simulink model "three_phase_motor"  (R2018a)
settings: Solver=VariableStepDiscrete  StartTime=0.0  StopTime=2  RelTol=1e-3
values from neighbouring files (symbols this model uses):
  Ts = 0.0001    [pump_ori_perf.mat]
libraries: powerlib x2, powerlib_meascontrol x2, electricdrivelib x1
settings Model: Creator=siwak  LastModifiedBy=siwak

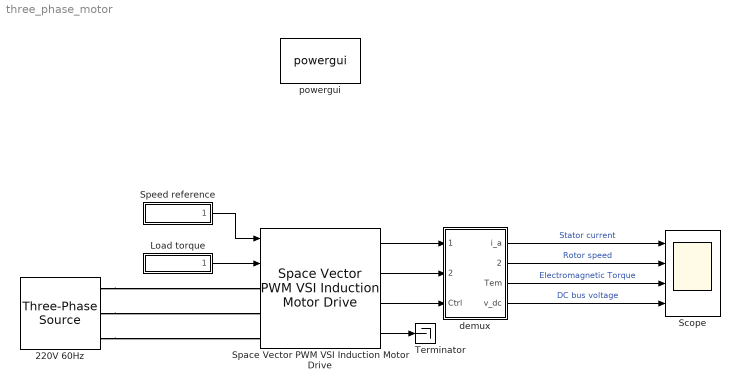
== system three_phase_motor ==
  220V 60Hz : powerlib/Electrical Sources/Three-Phase Source  InternalConnection=Yg  VoltagePhases=off  Voltage=220  PhaseAngle=0  Voltage_phases=[25e3 25e3 25e3]/sqrt(3)  PhaseAngles_phases=[0 -120 +120]  Frequency=60  NonIdealSource=on  SpecifyImpedance=off  Resistance=0.02  Inductance=0.05e-3  ShortCircuitLevel=100e6  BaseVoltage=25e3  XRratio=7  BusType=swing  Pref=0  Qref=0  Prefabc=[10e3, 10e3, 10e3]  Qrefabc=[0, 0, 0]  Qmin=-inf  Qmax=inf
  Load torque : Subsystem
  Scope : Scope  NumInputPorts=4
  Space Vector PWM VSI Induction Motor Drive : electricdrivelib/AC drives/Space Vector PWM VSI Induction Motor Drive  ReferenceFrame=Stationary  IterativeDiscreteModel=Trapezoidal non iterative  Pn=2238  Vn=220  fn=60  Rs=0.435  Lls=0.002  Lms=69.31e-3  Rr=0.816  Llr=0.002  ia=0  pha=0  ib=0  phb=0  ic=0  phc=0  J=0.089  Friction=0.005  p=2  slip=1  thdeg=0  Rsnb_rec=10e3  Csnb_rec=20e-9  Ron_rec=1e-3  Vf_rec=1.3  cap_bus=3400e-6  Rbrake=8  fbrake=4000  activationVoltage=340  shutdownVoltage=320  deviceType=IGBT / Diodes  Ron_inv=1e-3  Vf_inv=1.2  Vfd_inv=1.2  Tf=1e-6  Tt=2e-6  Tf_GTO=10e-6  Tt_GTO=20e-6  Rsnb_inv=500  Csnb_inv=1e-9  Acc=1800  Dec=-1800  kp_sc=9  ki_sc=10  fc_sc=100  Tsc=100e-6  ctrl_sat_min=-30  ctrl_sat_max=30  ctrl_f_min=0.05  ctrl_f_max=120  ctrl_v_min=10  ctrl_v_max=180  vh_ratio=3.2  zc_time=0.4  car_freq=4500  fc_bus=50  Tvect=20e-6  baseSampleTime=2e-06  outputBusMode=Multiple output buses  busLabels=off  MechanicalLoad=Torque Tm  modelDetailLevel=Detailed  driveType=AC2  AverageValue=off
      settings: SourceProductName=Simscape Power Systems  SourceProductBaseCode=PS
  Speed reference : Subsystem
  Terminator : Terminator
  demux : Subsystem
  powergui : powerlib/powergui  Priority=2  SimulationMode=Discrete  SampleTime=Ts  frequency=60  Iterations=50  frequencyindice=60  Pbase=100e6  ErrMax=1e-4  UnitsV=kV  UnitsW=MW  buscounter=0  FunctionMessages=off  echomessages=off  EnableUseOfTLC=off  CurrentSourceSwitches=off  DisableSnubberDevices=off  DisableRonSwitches=off  DisableVfSwitches=off  DisplayEquations=off  SolverType=Tustin/Backward Euler (TBE)  Interpol=off  ExternalGateDelay=off  methode=off  Ts=0  x0status=blocks  SPID=off  SwTol=0  HookPort=off  RestoreLinks=warning  ResistiveCurrentMeasurement=off  Frange=[0:2:500]  Ylog=off  Xlog=on  ShowGrid=off  save=off  variable=ZData  structure=0  ZoomFFT=on  StartTime=0.0  cycles=1  DisplayStyle=1  fundamental=60  FreqAxis=off  MaxFrequency=1000  frequencyindicesteady=1  RmsSteady=1  display=off
  wires:
  demux/3(Tem) -> Scope/3  "Electromagnetic Torque"
  Space Vector PWM VSI Induction Motor Drive/2 -> demux/2(Conv.)
  Space Vector PWM VSI Induction Motor Drive/3 -> demux/3(Ctrl)
  Space Vector PWM VSI Induction Motor Drive/4 -> Terminator/1
  Speed reference/1(" ") -> Space Vector PWM VSI Induction Motor Drive/1
  Space Vector PWM VSI Induction Motor Drive/1 -> demux/1(Motor)
  demux/2(speed) -> Scope/2  "Rotor speed"
  demux/4(v_dc) -> Scope/4  "DC bus voltage"
  Load torque/1(" ") -> Space Vector PWM VSI Induction Motor Drive/2
  demux/1(i_a) -> Scope/1  "Stator current"
  connections:
  220V 60Hz/RConn3 -- Space Vector PWM VSI Induction Motor Drive/LConn3
  220V 60Hz/RConn2 -- Space Vector PWM VSI Induction Motor Drive/LConn2
  220V 60Hz/RConn1 -- Space Vector PWM VSI Induction Motor Drive/LConn1

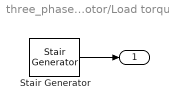
== system three_phase_motor/Load torque ==
  Stair Generator : powerlib_meascontrol/Pulse & Signal Generators/Stair Generator  t=[0 0.5 1.5]  e=[0 11 -11]  Ts=Ts
      settings: SourceProductName=Simscape Power Systems
  " " : Outport
  wires:
  Stair Generator/1 -> " "/1

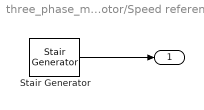
== system three_phase_motor/Speed reference ==
  Stair Generator : powerlib_meascontrol/Pulse & Signal Generators/Stair Generator  t=[0 1]  e=[1000 1500]  Ts=Ts
      settings: SourceProductName=Simscape Power Systems
  " " : Outport
  wires:
  Stair Generator/1 -> " "/1

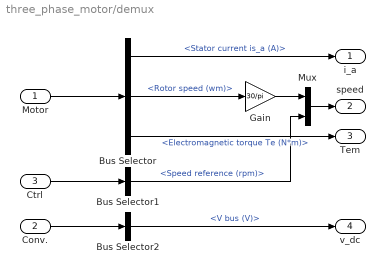
== system three_phase_motor/demux ==
  Motor : Inport
  Conv. : Inport  Port=2
  Ctrl : Inport  Port=3
  Bus Selector : BusSelector  OutputSignals=Stator measurements.Stator current is_a (A),Mechanical.Rotor speed (wm),Mechanical.Electromagnetic torque Te (N*m)
  Bus Selector1 : BusSelector  OutputSignals=Speed reference (rpm)
  Bus Selector2 : BusSelector  OutputSignals=V bus (V)
  Gain : Gain  Gain=30/pi  SaturateOnIntegerOverflow=on  OutDataTypeStr=Inherit: Same as input  ParamDataTypeStr=Inherit: Same as input
  Mux : Mux  Inputs=2
  i_a : Outport
  speed : Outport  Port=2
  Tem : Outport  Port=3
  v_dc : Outport  Port=4
  wires:
  Ctrl/1 -> Bus Selector1/1
  Gain/1 -> Mux/1
  Mux/1 -> speed/1
  Motor/1 -> Bus Selector/1
  Bus Selector/1 -> i_a/1  "<Stator current is_a (A)>"
  Bus Selector/2 -> Gain/1  "<Rotor speed (wm)>"
  Bus Selector/3 -> Tem/1  "<Electromagnetic torque Te (N*m)>"
  Bus Selector1/1 -> Mux/2  "<Speed reference (rpm)>"
  Conv./1 -> Bus Selector2/1
  Bus Selector2/1 -> v_dc/1  "<V bus (V)>"
